simulink model "multilevelinverter21"  (R2014b)
settings: Solver=ode45  StartTime=0.0  StopTime=0.2  MaxStep=.00001  RelTol=1e-3
libraries: powerlib x35, simulink x20
settings Model: Creator=Muruganandham  LastModifiedBy=SELVA
settings DataIOCC: SignalLoggingSaveFormat=ModelDataLogs
settings OptimizationCC: ExpressionDepthLimit=2147483647
settings DebuggingCC: UnderspecifiedInitializationDetection=Classic  MergeDetectMultiDrivingBlocksExec=none  FcnCallInpInsideContextMsg=UseLocalSettings  StateNameClashWarn=warning
settings GRTTargetCC: CombineOutputUpdateFcns=off  GRTInterface=on

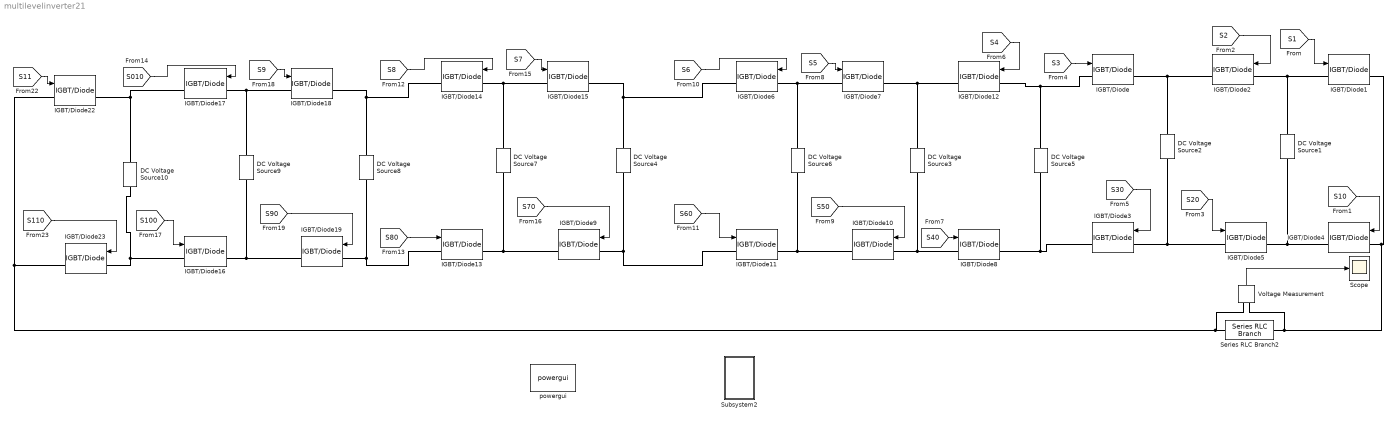
== system multilevelinverter21 ==
  DC Voltage Source{1..10} (10 alike) : powerlib/Electrical Sources/DC Voltage Source  Amplitude=32.8  Measurements=None
  IGBT/Diode{,1..19,22..23} (22 alike) : powerlib/Power Electronics/IGBT//Diode  Ron=1e-3  Rs=1e5  Cs=inf  Measurements=on
  Scope : Scope
      settings: YMin=-600  YMax=600  SaveName=bh
  Series RLC Branch2 : powerlib/Elements/Series RLC Branch  LConnTagsString=__new0  RConnTagsString=__new0  BranchType=R  Resistance=10  Inductance=1e-3  SetiL0=off  InitialCurrent=0  Capacitance=1e-6  Setx0=off  InitialVoltage=0  Measurements=None
  Subsystem2 : Subsystem  mask{fc=1000, m=1}
      mask prompts: fc "Switching frequency"; m "modulation index"
  Voltage Measurement : powerlib/Measurements/Voltage Measurement  PhasorSimulation=off  OutputType=Complex  PSBequivalent=0
  powergui : powerlib/powergui  Priority=1  SimulationMode=Discrete  SolverType=Tustin/Backward Euler (TBE)  SampleTime=50e-6  frequency=60  SPID=off  DisableSnubberDevices=off  DisableRonSwitches=off  DisableVfSwitches=off  SwTol=0  DisplayEquations=off  Interpol=off  methode=off  Ts=100  frequencyindice=0  Pbase=100e6  ErrMax=1e-4  Iterations=50  UnitsV=kV  UnitsW=MW  FunctionMessages=off  echomessages=off  HookPort=off  EnableUseOfTLC=off  x0status=blocks  RestoreLinks=warning  ResistiveCurrentMeasurement=off  Frange=[0:2:500]  Ylog=off  Xlog=on  ShowGrid=off  save=off  variable=ZData  structure=bh  ZoomFFT=off  StartTime=0.0  cycles=1  DisplayStyle=1  fundamental=50  FreqAxis=off  MaxFrequency=1000  frequencyindicesteady=1  RmsSteady=1  display=off
  wires:
  [S1] -> IGBT/Diode1/1
  [S10] -> IGBT/Diode4/1
  [S2] -> IGBT/Diode2/1
  [S20] -> IGBT/Diode5/1
  [S3] -> IGBT/Diode/1
  [S30] -> IGBT/Diode3/1
  [S40] -> IGBT/Diode8/1
  [S6] -> IGBT/Diode6/1
  [S4] -> IGBT/Diode12/1
  [S5] -> IGBT/Diode7/1
  [S50] -> IGBT/Diode10/1
  [S60] -> IGBT/Diode11/1
  [S8] -> IGBT/Diode14/1
  [S7] -> IGBT/Diode15/1
  [S70] -> IGBT/Diode9/1
  [S80] -> IGBT/Diode13/1
  [S010] -> IGBT/Diode17/1
  [S9] -> IGBT/Diode18/1
  [S90] -> IGBT/Diode19/1
  [S100] -> IGBT/Diode16/1
  [S11] -> IGBT/Diode22/1
  [S110] -> IGBT/Diode23/1
  Voltage Measurement/1 -> Scope/1
  connections:
  DC Voltage Source2/LConn1 -- IGBT/Diode/RConn1 -- IGBT/Diode2/RConn1
  DC Voltage Source1/RConn1 -- IGBT/Diode2/LConn1 -- IGBT/Diode1/LConn1
  DC Voltage Source2/RConn1 -- IGBT/Diode3/LConn1 -- IGBT/Diode5/LConn1
  DC Voltage Source1/LConn1 -- IGBT/Diode5/RConn1 -- IGBT/Diode4/RConn1
  IGBT/Diode1/RConn1 -- Voltage Measurement/LConn2 -- Series RLC Branch2/RConn1 -- IGBT/Diode4/LConn1
  DC Voltage Source6/RConn1 -- IGBT/Diode6/LConn1 -- IGBT/Diode7/LConn1
  DC Voltage Source3/LConn1 -- IGBT/Diode7/RConn1 -- IGBT/Diode12/RConn1
  DC Voltage Source6/LConn1 -- IGBT/Diode11/RConn1 -- IGBT/Diode10/RConn1
  DC Voltage Source3/RConn1 -- IGBT/Diode10/LConn1 -- IGBT/Diode8/LConn1
  IGBT/Diode/LConn1 -- IGBT/Diode12/LConn1 -- DC Voltage Source5/RConn1
  IGBT/Diode3/RConn1 -- IGBT/Diode8/RConn1 -- DC Voltage Source5/LConn1
  IGBT/Diode15/LConn1 -- DC Voltage Source7/RConn1 -- IGBT/Diode14/LConn1
  IGBT/Diode15/RConn1 -- DC Voltage Source4/LConn1 -- IGBT/Diode6/RConn1
  IGBT/Diode9/RConn1 -- DC Voltage Source7/LConn1 -- IGBT/Diode13/RConn1
  IGBT/Diode9/LConn1 -- IGBT/Diode11/LConn1 -- DC Voltage Source4/RConn1
  IGBT/Diode18/LConn1 -- DC Voltage Source9/RConn1 -- IGBT/Diode17/LConn1
  IGBT/Diode18/RConn1 -- DC Voltage Source8/LConn1 -- IGBT/Diode14/RConn1
  IGBT/Diode19/RConn1 -- DC Voltage Source9/LConn1 -- IGBT/Diode16/RConn1
  DC Voltage Source8/RConn1 -- IGBT/Diode13/LConn1 -- IGBT/Diode19/LConn1
  IGBT/Diode22/RConn1 -- IGBT/Diode17/RConn1 -- DC Voltage Source10/LConn1
  DC Voltage Source10/RConn1 -- IGBT/Diode23/LConn1 -- IGBT/Diode16/LConn1
  IGBT/Diode23/RConn1 -- Voltage Measurement/LConn1 -- Series RLC Branch2/LConn1 -- IGBT/Diode22/LConn1

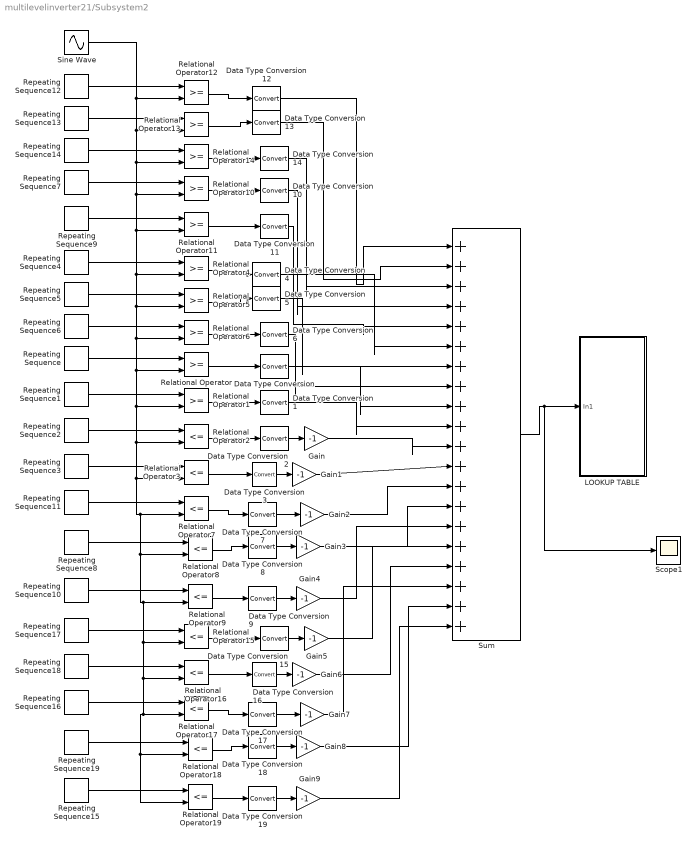
== system multilevelinverter21/Subsystem2 ==
  Data Type Conversion{,1..19} (20 alike) : DataTypeConversion
  Gain{,1..9} (10 alike) : Gain  Gain=-1
  LOOKUP TABLE : Subsystem
  Relational Operator{,1,4..6,10..14} (10 alike) : RelationalOperator  OutDataTypeStr=boolean
  Relational Operator{2..3,7..9,15..19} (10 alike) : RelationalOperator  Operator=<=  OutDataTypeStr=boolean
  Repeating Sequence : simulink/Sources/Repeating Sequence  rep_seq_t="[0 (1/fc)/2  (1/fc)]"  rep_seq_y=[2 1 2]
  Repeating Sequence1 : simulink/Sources/Repeating Sequence  rep_seq_t="[0 (1/fc)/2  (1/fc)]"  rep_seq_y=[1 0 1]
  Repeating Sequence10 : simulink/Sources/Repeating Sequence  rep_seq_t="[0 (1/fc)/2  (1/fc)]"  rep_seq_y=[-5 -4 -5]
  Repeating Sequence11 : simulink/Sources/Repeating Sequence  rep_seq_t="[0 (1/fc)/2  (1/fc)]"  rep_seq_y=[-3 -2 -3]
  Repeating Sequence12 : simulink/Sources/Repeating Sequence  rep_seq_t="[0 (1/fc)/2  (1/fc)]"  rep_seq_y=[9 10 9]
  Repeating Sequence13 : simulink/Sources/Repeating Sequence  rep_seq_t="[0 (1/fc)/2  (1/fc)]"  rep_seq_y=[9 8 9]
  Repeating Sequence14 : simulink/Sources/Repeating Sequence  rep_seq_t="[0 (1/fc)/2  (1/fc)]"  rep_seq_y=[8 7 8]
  Repeating Sequence15 : simulink/Sources/Repeating Sequence  rep_seq_t="[0 (1/fc)/2  (1/fc)]"  rep_seq_y=[-10 -9 -10]
  Repeating Sequence16 : simulink/Sources/Repeating Sequence  rep_seq_t="[0 (1/fc)/2  (1/fc)]"  rep_seq_y=[-8 -7 -8]
  Repeating Sequence17 : simulink/Sources/Repeating Sequence  rep_seq_t="[0 (1/fc)/2  (1/fc)]"  rep_seq_y=[-6 -5 -6]
  Repeating Sequence18 : simulink/Sources/Repeating Sequence  rep_seq_t="[0 (1/fc)/2  (1/fc)]"  rep_seq_y=[-7 -6 -7]
  Repeating Sequence19 : simulink/Sources/Repeating Sequence  rep_seq_t="[0 (1/fc)/2  (1/fc)]"  rep_seq_y=[-9 -8 -9]
  Repeating Sequence2 : simulink/Sources/Repeating Sequence  rep_seq_t="[0 (1/fc)/2  (1/fc)]"  rep_seq_y=[-1 0 -1]
  Repeating Sequence3 : simulink/Sources/Repeating Sequence  rep_seq_t="[0 (1/fc)/2  (1/fc)]"  rep_seq_y=[-2 -1 -2]
  Repeating Sequence4 : simulink/Sources/Repeating Sequence  rep_seq_t="[0 (1/fc)/2  (1/fc)]"  rep_seq_y=[5 4 5]
  Repeating Sequence5 : simulink/Sources/Repeating Sequence  rep_seq_t="[0 (1/fc)/2  (1/fc)]"  rep_seq_y=[4 3 4]
  Repeating Sequence6 : simulink/Sources/Repeating Sequence  rep_seq_t="[0 (1/fc)/2  (1/fc)]"  rep_seq_y=[3 2 3]
  Repeating Sequence7 : simulink/Sources/Repeating Sequence  rep_seq_t="[0 (1/fc)/2  (1/fc)]"  rep_seq_y=[7 6 7]
  Repeating Sequence8 : simulink/Sources/Repeating Sequence  rep_seq_t="[0 (1/fc)/2  (1/fc)]"  rep_seq_y=[-4 -3 -4]
  Repeating Sequence9 : simulink/Sources/Repeating Sequence  rep_seq_t="[0 (1/fc)/2  (1/fc)]"  rep_seq_y=[6 5 6]
  Scope1 : Scope
      settings: YMin=-600  YMax=600  SaveName=bh2
  Sine Wave : Sin  Amplitude=10*m  Frequency=2*pi*50  SampleTime=0
  Sum : Sum  Inputs=|++++++++++++++++++++
  wires:
  Data Type Conversion3/1 -> Gain1/1
  Data Type Conversion2/1 -> Gain/1
  Relational Operator3/1 -> Data Type Conversion3/1
  Relational Operator2/1 -> Data Type Conversion2/1
  Repeating Sequence3/1 -> Relational Operator3/1
  Repeating Sequence2/1 -> Relational Operator2/1
  Repeating Sequence1/1 -> Relational Operator1/1
  Repeating Sequence/1 -> Relational Operator/1
  Relational Operator1/1 -> Data Type Conversion1/1
  Relational Operator/1 -> Data Type Conversion/1
  Repeating Sequence6/1 -> Relational Operator6/1
  Repeating Sequence5/1 -> Relational Operator5/1
  Repeating Sequence4/1 -> Relational Operator4/1
  Relational Operator6/1 -> Data Type Conversion6/1
  Relational Operator5/1 -> Data Type Conversion5/1
  Relational Operator4/1 -> Data Type Conversion4/1
  Repeating Sequence8/1 -> Relational Operator8/1
  Repeating Sequence11/1 -> Relational Operator7/1
  Relational Operator9/1 -> Data Type Conversion9/1
  Relational Operator8/1 -> Data Type Conversion8/1
  Relational Operator7/1 -> Data Type Conversion7/1
  Data Type Conversion9/1 -> Gain4/1
  Data Type Conversion8/1 -> Gain3/1
  Data Type Conversion7/1 -> Gain2/1
  Repeating Sequence10/1 -> Relational Operator9/1
  Sum/1 -> Scope1/1, LOOKUP TABLE/1(In1)
  Repeating Sequence9/1 -> Relational Operator11/1
  Repeating Sequence7/1 -> Relational Operator10/1
  Relational Operator11/1 -> Data Type Conversion11/1
  Relational Operator10/1 -> Data Type Conversion10/1
  Repeating Sequence14/1 -> Relational Operator14/1
  Repeating Sequence13/1 -> Relational Operator13/1
  Repeating Sequence12/1 -> Relational Operator12/1
  Relational Operator14/1 -> Data Type Conversion14/1
  Relational Operator13/1 -> Data Type Conversion13/1
  Relational Operator12/1 -> Data Type Conversion12/1
  Data Type Conversion16/1 -> Gain6/1
  Data Type Conversion15/1 -> Gain5/1
  Relational Operator16/1 -> Data Type Conversion16/1
  Relational Operator15/1 -> Data Type Conversion15/1
  Repeating Sequence18/1 -> Relational Operator16/1
  Repeating Sequence17/1 -> Relational Operator15/1
  Repeating Sequence19/1 -> Relational Operator18/1
  Repeating Sequence16/1 -> Relational Operator17/1
  Relational Operator19/1 -> Data Type Conversion19/1
  Relational Operator18/1 -> Data Type Conversion18/1
  Relational Operator17/1 -> Data Type Conversion17/1
  Data Type Conversion19/1 -> Gain9/1
  Data Type Conversion18/1 -> Gain8/1
  Data Type Conversion17/1 -> Gain7/1
  Repeating Sequence15/1 -> Relational Operator19/1
  Sine Wave/1 -> Relational Operator12/2, Relational Operator13/2, Relational Operator14/2, Relational Operator10/2, Relational Operator11/2, Relational Operator5/2, Relational Operator6/2, Relational Operator/2, Relational Operator1/2, Relational Operator2/2, Relational Operator3/2, Relational Operator7/2, Relational Operator18/2, Relational Operator19/2, Relational Operator17/2, Relational Operator16/2, Relational Operator15/2, Relational Operator9/2, Relational Operator8/2, Relational Operator4/2
  Data Type Conversion12/1 -> Sum/1
  Data Type Conversion13/1 -> Sum/2
  Data Type Conversion14/1 -> Sum/3
  Data Type Conversion10/1 -> Sum/4
  Data Type Conversion11/1 -> Sum/5
  Data Type Conversion4/1 -> Sum/6
  Data Type Conversion5/1 -> Sum/7
  Data Type Conversion6/1 -> Sum/8
  Data Type Conversion/1 -> Sum/9
  Data Type Conversion1/1 -> Sum/10
  Gain/1 -> Sum/11
  Gain1/1 -> Sum/12
  Gain2/1 -> Sum/13
  Gain3/1 -> Sum/14
  Gain4/1 -> Sum/15
  Gain5/1 -> Sum/16
  Gain6/1 -> Sum/17
  Gain7/1 -> Sum/18
  Gain8/1 -> Sum/19
  Gain9/1 -> Sum/20

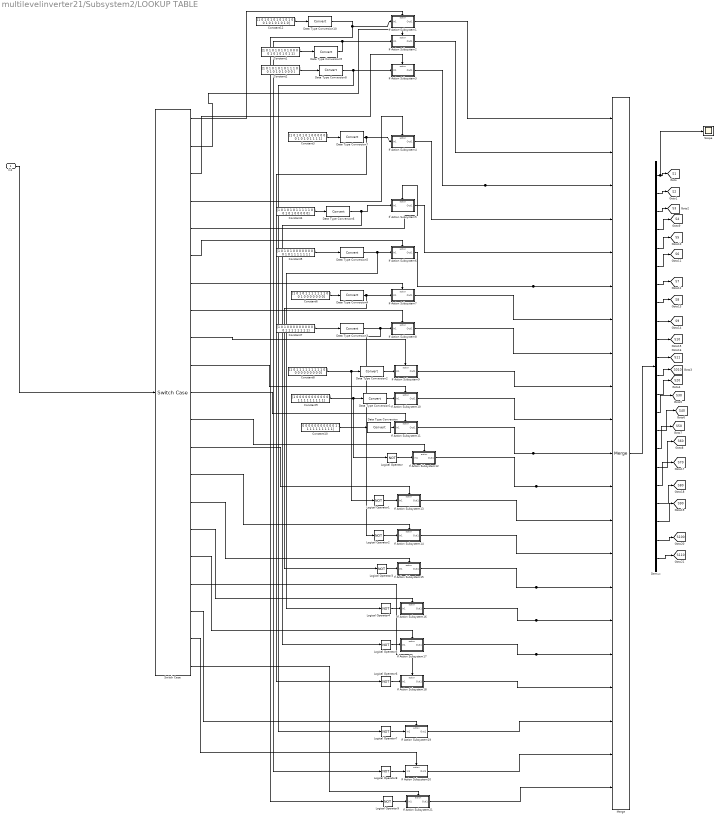
== system multilevelinverter21/Subsystem2/LOOKUP TABLE ==
  In1 : Inport
  Constant1 : Constant  Value=[1 0 1 0 1 0 1 0 1 0 0 0 1 0 1 0 1 0 1 0 1 1]
  Constant10 : Constant  Value=[0 0 0 0 0 0 0 0 0 0 0 1 1 1 1 1 1 1 1 1 1 1]
  Constant12 : Constant  Value=[1 0 1 0 1 0 1 0 1 0 1 0 1 0 1 0 1 0 1 0 1 0]
  Constant2 : Constant  Value=[1 0 1 0 1 0 1 0 1 1 1 0 1 0 1 0 1 0 1 0 0 0 ]
  Constant3 : Constant  Value=[1 0 1 0 1 0 1 0 0 0 0 0 1 0 1 0 1 0 1 1 1 1]
  Constant4 : Constant  Value=[1 0 1 0 1 0 1 1 1 1 1 0 1 0 1 0 1 0 0 0 0 0]
  Constant5 : Constant  Value=[1 0 1 0 1 0 0 0 0 0 0 0 1 0 1 0 1 1 1 1 1 1 ]
  Constant6 : Constant  Value=[1 0 1 0 1 1 1 1 1 1 1 0 1 0 1 0 0 0 0 0 0 0]
  Constant7 : Constant  Value=[1 0 1 0 0 0 0 0 0 0 0 0 1 0 1 1 1 1 1 1 1 1]
  Constant8 : Constant  Value=[1 0 1 1 1 1 1 1 1 1 1 0 1 0 0 0 0 0 0 0 0 0]
  Constant9 : Constant  Value=[1 0 0 0 0 0 0 0 0 0 0 0 1 1 1 1 1 1 1 1 1 1]
  Data Type Conversion{,1..10} (11 alike) : DataTypeConversion
  Demux : Demux  Outputs=22
  If Action Subsystem1 : Subsystem  TreatAsAtomicUnit=on
  If Action Subsystem10 : Subsystem  TreatAsAtomicUnit=on
  If Action Subsystem11 : Subsystem  TreatAsAtomicUnit=on
  If Action Subsystem12 : Subsystem  TreatAsAtomicUnit=on
  If Action Subsystem13 : Subsystem  TreatAsAtomicUnit=on
  If Action Subsystem14 : Subsystem  TreatAsAtomicUnit=on
  If Action Subsystem15 : Subsystem  TreatAsAtomicUnit=on
  If Action Subsystem16 : Subsystem  TreatAsAtomicUnit=on
  If Action Subsystem17 : Subsystem  TreatAsAtomicUnit=on
  If Action Subsystem18 : Subsystem  TreatAsAtomicUnit=on
  If Action Subsystem19 : Subsystem  TreatAsAtomicUnit=on
  If Action Subsystem2 : Subsystem  TreatAsAtomicUnit=on
  If Action Subsystem20 : Subsystem  TreatAsAtomicUnit=on
  If Action Subsystem21 : Subsystem  TreatAsAtomicUnit=on
  If Action Subsystem3 : Subsystem  TreatAsAtomicUnit=on
  If Action Subsystem4 : Subsystem  TreatAsAtomicUnit=on
  If Action Subsystem5 : Subsystem  TreatAsAtomicUnit=on
  If Action Subsystem6 : Subsystem  TreatAsAtomicUnit=on
  If Action Subsystem7 : Subsystem  TreatAsAtomicUnit=on
  If Action Subsystem8 : Subsystem  TreatAsAtomicUnit=on
  If Action Subsystem9 : Subsystem  TreatAsAtomicUnit=on
  Logical Operator{,1..9} (10 alike) : Logic  Operator=NOT  AllPortsSameDT=off  OutDataTypeStr=boolean
  Merge : Merge  Inputs=21  AllowUnequalInputPortWidths=on
  Scope : Scope
      settings: YMin=-1  YMax=1
  Switch Case : SwitchCase  CaseConditions={10 9 8 7 6 5 4 3 2 1 0 -1 -2 -3 -4 -5 -6 -7 -8 -9 -10}  ShowDefaultCase=off
  tag scope: S010=global, S100=global, S10=global, S110=global, S11=global, S1=global, S20=global, S2=global, S30=global, S3=global, S40=global, S4=global, S50=global, S5=global, S60=global, S6=global, S70=global, S7=global, S80=global, S8=global, S90=global, S9=global
  wires:
  Merge/1 -> Demux/1
  In1/1 -> Switch Case/1
  Constant12/1 -> Data Type Conversion10/1
  Switch Case/1 -> If Action Subsystem1/Action
  Switch Case/2 -> If Action Subsystem2/Action
  Constant1/1 -> Data Type Conversion9/1
  Constant2/1 -> Data Type Conversion8/1
  Switch Case/3 -> If Action Subsystem3/Action
  Switch Case/4 -> If Action Subsystem4/Action
  Constant3/1 -> Data Type Conversion7/1
  Constant4/1 -> Data Type Conversion6/1
  Switch Case/5 -> If Action Subsystem5/Action
  Switch Case/6 -> If Action Subsystem6/Action
  Constant5/1 -> Data Type Conversion5/1
  Constant6/1 -> Data Type Conversion4/1
  Switch Case/7 -> If Action Subsystem7/Action
  Constant7/1 -> Data Type Conversion3/1
  Switch Case/8 -> If Action Subsystem8/Action
  Constant8/1 -> Data Type Conversion2/1, Logical Operator1/1
  Switch Case/9 -> If Action Subsystem9/Action
  Constant9/1 -> Logical Operator/1, Data Type Conversion1/1
  Switch Case/10 -> If Action Subsystem10/Action
  Constant10/1 -> Data Type Conversion/1
  Switch Case/11 -> If Action Subsystem11/Action
  Logical Operator/1 -> If Action Subsystem12/1(In1)
  Switch Case/12 -> If Action Subsystem12/Action
  Switch Case/13 -> If Action Subsystem13/Action
  Logical Operator1/1 -> If Action Subsystem13/1(In1)
  Switch Case/14 -> If Action Subsystem14/Action
  Logical Operator2/1 -> If Action Subsystem14/1(In1)
  Logical Operator3/1 -> If Action Subsystem15/1(In1)
  Switch Case/15 -> If Action Subsystem15/Action
  Switch Case/16 -> If Action Subsystem16/Action
  Logical Operator4/1 -> If Action Subsystem16/1(In1)
  Switch Case/17 -> If Action Subsystem17/Action
  Logical Operator5/1 -> If Action Subsystem17/1(In1)
  Switch Case/18 -> If Action Subsystem18/Action
  Logical Operator6/1 -> If Action Subsystem18/1(In1)
  Switch Case/19 -> If Action Subsystem19/Action
  Logical Operator7/1 -> If Action Subsystem19/1(In1)
  Switch Case/20 -> If Action Subsystem20/Action
  Logical Operator8/1 -> If Action Subsystem20/1(In1)
  If Action Subsystem21/1(Out1) -> Merge/21
  Switch Case/21 -> If Action Subsystem21/Action
  Logical Operator9/1 -> If Action Subsystem21/1(In1)
  Demux/2 -> [S2]
  Demux/3 -> [S3]
  Demux/4 -> [S4]
  Demux/5 -> [S5]
  Demux/6 -> [S6]
  Demux/12 -> [S010]
  Demux/7 -> [S7]
  Demux/8 -> [S8]
  Demux/9 -> [S9]
  Demux/10 -> [S10]
  Demux/11 -> [S11]
  Demux/13 -> [S20]
  Demux/14 -> [S30]
  Demux/15 -> [S40]
  Demux/16 -> [S50]
  Demux/17 -> [S60]
  Demux/18 -> [S70]
  Demux/19 -> [S80]
  Demux/20 -> [S90]
  Demux/21 -> [S100]
  Demux/22 -> [S110]
  If Action Subsystem1/1(Out1) -> Merge/1
  If Action Subsystem2/1(Out1) -> Merge/2
  If Action Subsystem3/1(Out1) -> Merge/3
  If Action Subsystem4/1(Out1) -> Merge/4
  If Action Subsystem5/1(Out1) -> Merge/5
  If Action Subsystem6/1(Out1) -> Merge/6
  If Action Subsystem7/1(Out1) -> Merge/7
  If Action Subsystem8/1(Out1) -> Merge/8
  If Action Subsystem9/1(Out1) -> Merge/9
  If Action Subsystem10/1(Out1) -> Merge/10
  If Action Subsystem11/1(Out1) -> Merge/11
  If Action Subsystem12/1(Out1) -> Merge/12
  If Action Subsystem13/1(Out1) -> Merge/13
  If Action Subsystem14/1(Out1) -> Merge/14
  If Action Subsystem15/1(Out1) -> Merge/15
  If Action Subsystem16/1(Out1) -> Merge/16
  If Action Subsystem17/1(Out1) -> Merge/17
  If Action Subsystem18/1(Out1) -> Merge/18
  If Action Subsystem19/1(Out1) -> Merge/19
  If Action Subsystem20/1(Out1) -> Merge/20
  Demux/1 -> Scope/1, [S1]
  Data Type Conversion/1 -> If Action Subsystem11/1(In1)
  Data Type Conversion1/1 -> If Action Subsystem10/1(In1)
  Data Type Conversion2/1 -> If Action Subsystem9/1(In1)
  Data Type Conversion3/1 -> Logical Operator2/1, If Action Subsystem8/1(In1)
  Data Type Conversion4/1 -> Logical Operator3/1, If Action Subsystem7/1(In1)
  Data Type Conversion5/1 -> Logical Operator4/1, If Action Subsystem6/1(In1)
  Data Type Conversion6/1 -> Logical Operator5/1, If Action Subsystem5/1(In1)
  Data Type Conversion7/1 -> Logical Operator6/1, If Action Subsystem4/1(In1)
  Data Type Conversion8/1 -> Logical Operator7/1, If Action Subsystem3/1(In1)
  Data Type Conversion9/1 -> If Action Subsystem2/1(In1), Logical Operator8/1
  Data Type Conversion10/1 -> Logical Operator9/1, If Action Subsystem1/1(In1)

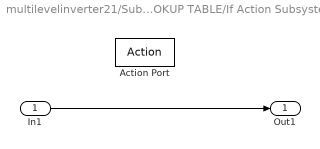
== system multilevelinverter21/Subsystem2/LOOKUP TABLE/If Action Subsystem1 ==
  In1 : Inport
  Action Port : ActionPort  ActionType=case
  Out1 : Outport
  wires:
  In1/1 -> Out1/1

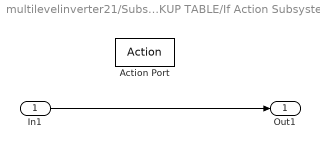
== system multilevelinverter21/Subsystem2/LOOKUP TABLE/If Action Subsystem10 ==
  In1 : Inport
  Action Port : ActionPort  ActionType=case
  Out1 : Outport
  wires:
  In1/1 -> Out1/1

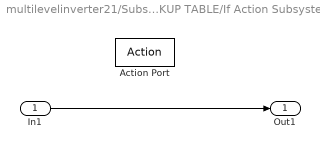
== system multilevelinverter21/Subsystem2/LOOKUP TABLE/If Action Subsystem11 ==
  In1 : Inport
  Action Port : ActionPort  ActionType=case
  Out1 : Outport
  wires:
  In1/1 -> Out1/1

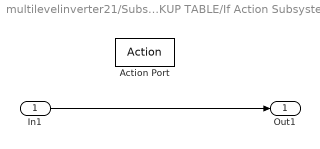
== system multilevelinverter21/Subsystem2/LOOKUP TABLE/If Action Subsystem12 ==
  In1 : Inport
  Action Port : ActionPort  ActionType=case
  Out1 : Outport
  wires:
  In1/1 -> Out1/1

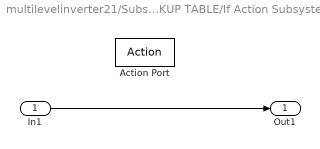
== system multilevelinverter21/Subsystem2/LOOKUP TABLE/If Action Subsystem13 ==
  In1 : Inport
  Action Port : ActionPort  ActionType=case
  Out1 : Outport
  wires:
  In1/1 -> Out1/1

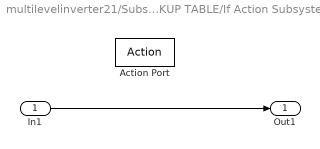
== system multilevelinverter21/Subsystem2/LOOKUP TABLE/If Action Subsystem14 ==
  In1 : Inport
  Action Port : ActionPort  ActionType=case
  Out1 : Outport
  wires:
  In1/1 -> Out1/1

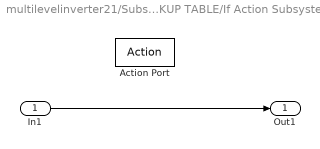
== system multilevelinverter21/Subsystem2/LOOKUP TABLE/If Action Subsystem15 ==
  In1 : Inport
  Action Port : ActionPort  ActionType=case
  Out1 : Outport
  wires:
  In1/1 -> Out1/1

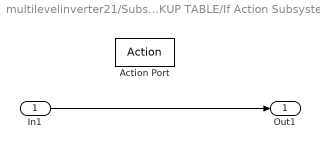
== system multilevelinverter21/Subsystem2/LOOKUP TABLE/If Action Subsystem16 ==
  In1 : Inport
  Action Port : ActionPort  ActionType=case
  Out1 : Outport
  wires:
  In1/1 -> Out1/1

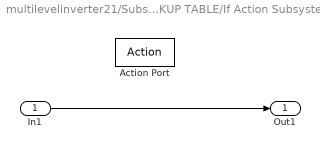
== system multilevelinverter21/Subsystem2/LOOKUP TABLE/If Action Subsystem17 ==
  In1 : Inport
  Action Port : ActionPort  ActionType=case
  Out1 : Outport
  wires:
  In1/1 -> Out1/1

== system multilevelinverter21/Subsystem2/LOOKUP TABLE/If Action Subsystem18 ==
  In1 : Inport
  Action Port : ActionPort  ActionType=case
  Out1 : Outport
  wires:
  In1/1 -> Out1/1

== system multilevelinverter21/Subsystem2/LOOKUP TABLE/If Action Subsystem19 ==
  In1 : Inport
  Action Port : ActionPort  ActionType=case
  Out1 : Outport
  wires:
  In1/1 -> Out1/1

== system multilevelinverter21/Subsystem2/LOOKUP TABLE/If Action Subsystem2 ==
  In1 : Inport
  Action Port : ActionPort  ActionType=case
  Out1 : Outport
  wires:
  In1/1 -> Out1/1

== system multilevelinverter21/Subsystem2/LOOKUP TABLE/If Action Subsystem20 ==
  In1 : Inport
  Action Port : ActionPort  ActionType=case
  Out1 : Outport
  wires:
  In1/1 -> Out1/1

== system multilevelinverter21/Subsystem2/LOOKUP TABLE/If Action Subsystem21 ==
  In1 : Inport
  Action Port : ActionPort  ActionType=case
  Out1 : Outport
  wires:
  In1/1 -> Out1/1

== system multilevelinverter21/Subsystem2/LOOKUP TABLE/If Action Subsystem3 ==
  In1 : Inport
  Action Port : ActionPort  ActionType=case
  Out1 : Outport
  wires:
  In1/1 -> Out1/1

== system multilevelinverter21/Subsystem2/LOOKUP TABLE/If Action Subsystem4 ==
  In1 : Inport
  Action Port : ActionPort  ActionType=case
  Out1 : Outport
  wires:
  In1/1 -> Out1/1

== system multilevelinverter21/Subsystem2/LOOKUP TABLE/If Action Subsystem5 ==
  In1 : Inport
  Action Port : ActionPort  ActionType=case
  Out1 : Outport
  wires:
  In1/1 -> Out1/1

== system multilevelinverter21/Subsystem2/LOOKUP TABLE/If Action Subsystem6 ==
  In1 : Inport
  Action Port : ActionPort  ActionType=case
  Out1 : Outport
  wires:
  In1/1 -> Out1/1

== system multilevelinverter21/Subsystem2/LOOKUP TABLE/If Action Subsystem7 ==
  In1 : Inport
  Action Port : ActionPort  ActionType=case
  Out1 : Outport
  wires:
  In1/1 -> Out1/1

== system multilevelinverter21/Subsystem2/LOOKUP TABLE/If Action Subsystem8 ==
  In1 : Inport
  Action Port : ActionPort  ActionType=case
  Out1 : Outport
  wires:
  In1/1 -> Out1/1

== system multilevelinverter21/Subsystem2/LOOKUP TABLE/If Action Subsystem9 ==
  In1 : Inport
  Action Port : ActionPort  ActionType=case
  Out1 : Outport
  wires:
  In1/1 -> Out1/1
